simulink model "DDCU_wxt_v02_forA_LabviewV02"  (R2014a)
settings: Solver=FixedStepDiscrete  StartTime=0.0  StopTime=50  FixedStep=0.0005  RelTol=1e-3
InitFcn:
  | Veh_Par_wxt
values from neighbouring files (symbols this model uses):
  ag_thr = 0.4*g    (= 3.924)    [Veh_Par_wxt.m]
  B = 2.25    [Veh_Par_wxt.m]
  bra_pre_em = 12    [Veh_Par_wxt.m]
  bra_pre_gz2 = 12/3    (= 4)    [Veh_Par_wxt.m]
  bra_pre_gz34 = 12/3    (= 4)    [Veh_Par_wxt.m]
  bra_pre_yd = 12/2    (= 6)    [Veh_Par_wxt.m]
  brakepre_dem_data = [0 1 2 3 4 5 6 7 8 9 10 11 12]    [Veh_Par_wxt.m]
  brakeTrq_dem_data = [0 218.198 436.396 654.594 872.792 1090.99 1309.188 1527.386 1745.584 1963.782 2181.98 2400.178 2618.376]    [Veh_Par_wxt.m]
  bratrq_max = 4*2618.376    (= 10473.504)    [Veh_Par_wxt.m]
  eff_tran = 0.75    [Veh_Par_wxt.m]
  G = Mass*g    (= 36297)    [Veh_Par_wxt.m]
  kd1 = 1    [Veh_Par_wxt.m]
  kd2 = 1    [Veh_Par_wxt.m]
  kd3 = 1    [Veh_Par_wxt.m]
  ki1 = 1    [Veh_Par_wxt.m]
  ki2 = 1    [Veh_Par_wxt.m]
  ki3 = 1    [Veh_Par_wxt.m]
  kp1 = 1    [Veh_Par_wxt.m]
  kp2 = 1    [Veh_Par_wxt.m]
  kp3 = 1    [Veh_Par_wxt.m]
  L = 3.12    [Veh_Par_wxt.m]
  premax = 12    [Veh_Par_wxt.m]
  Radius = 0.20    (= 0.2)    [Veh_Par_wxt.m]
  s_opt_yi_add = 0.05    [Veh_Par_wxt.m]
  s_opt_zhuan_add = 0.05    [Veh_Par_wxt.m]
  spd_map_mot = [0 100 200 300 360 400 500 600 700 800 900]*tras_ratio    [Veh_Par_wxt.m]
  spdmax = 900*tras_ratio    (= 5580)    [Veh_Par_wxt.m]
  speed_thr_park = 5/3.6/Radius*30/pi    (= 66.3145596216)    [Veh_Par_wxt.m]
  tras_ratio = 6.2    [Veh_Par_wxt.m]
  trq_map_mot = [1200 1200 1200 1200 1200 1080 864 720 617 540 480]/tras_ratio    [Veh_Par_wxt.m]
  trqmax = 80    [Veh_Par_wxt.m]
  v_thr1_b = 5    [Veh_Par_wxt.m]
  v_thr2_b = 20    [Veh_Par_wxt.m]
  v_thr_park = 5    [Veh_Par_wxt.m]
undefined symbols (not defined in the file or in its folder): DiscIntNeverNeededParam
libraries: simulink x231, ec5744lib x19
(part 5 of 16)

== system DDCU_wxt_v02_forA_LabviewV02/Data_Input/MCU2_VCU3/MCU2_VCU3 ==
  input : Inport
  Enable : EnablePort
  Demux : Demux  Outputs=8
  M4Current_Ad : Sum
  M4Current_Convert : DataTypeConversion  OutDataTypeStr=uint32
  M4Current_F : Gain  Gain=0.5
  M4Current_L : simulink/Logic and Bit Operations/Bitwise Operator  logicop=AND  UseBitMask=on  BitMask=65520  BitMaskRealWorld=Stored Integer
  M4Current_O : Constant  Value=-600  OutDataTypeStr=single
  M4Current_S : ArithShift  BitShiftNumber=4
  M4Current_Sub : Subsystem
  M4Current_sat : Saturate  UpperLimit=1447.5  LowerLimit=-600
  M4Currentcv : DataTypeConversion
  M4Currentinput3_Ad : Sum
  M4Currentinput3_C : Constant  Value=256
  M4Currentinput3_P : Product
  M4Direction_Ad : Sum
  M4Direction_Convert : DataTypeConversion  OutDataTypeStr=uint32
  M4Direction_F : Gain
  M4Direction_L : simulink/Logic and Bit Operations/Bitwise Operator  logicop=AND  UseBitMask=on  BitMask=128  BitMaskRealWorld=Stored Integer
  M4Direction_O : Constant  Value=0  OutDataTypeStr=single
  M4Direction_S : ArithShift  BitShiftNumber=7
  M4Direction_Sub : Subsystem
  M4Direction_sat : Saturate  UpperLimit=1  LowerLimit=0
  M4Directioncv : DataTypeConversion
  M4HeartBeat_Ad : Sum
  M4HeartBeat_Convert : DataTypeConversion  OutDataTypeStr=uint32
  M4HeartBeat_F : Gain
  M4HeartBeat_L : simulink/Logic and Bit Operations/Bitwise Operator  logicop=AND  UseBitMask=on  BitMask=15  BitMaskRealWorld=Stored Integer
  M4HeartBeat_O : Constant  Value=0  OutDataTypeStr=single
  M4HeartBeat_S : ArithShift
  M4HeartBeat_Sub : Subsystem
  M4HeartBeat_sat : Saturate  UpperLimit=15  LowerLimit=0
  M4HeartBeatcv : DataTypeConversion
  M4InputVolt_Ad : Sum
  M4InputVolt_Convert : DataTypeConversion  OutDataTypeStr=uint32
  M4InputVolt_F : Gain  Gain=0.25
  M4InputVolt_L : simulink/Logic and Bit Operations/Bitwise Operator  logicop=AND  UseBitMask=on  BitMask=4095  BitMaskRealWorld=Stored Integer
  M4InputVolt_O : Constant  Value=0  OutDataTypeStr=single
  M4InputVolt_S : ArithShift
  M4InputVolt_Sub : Subsystem
  M4InputVolt_sat : Saturate  UpperLimit=1023.75  LowerLimit=0
  M4InputVoltcv : DataTypeConversion
  M4InputVoltinput8_Ad : Sum
  M4InputVoltinput8_C : Constant  Value=256
  M4InputVoltinput8_P : Product
  M4Speed_Ad : Sum
  M4Speed_Convert : DataTypeConversion  OutDataTypeStr=uint32
  M4Speed_F : Gain  Gain=5
  M4Speed_L : simulink/Logic and Bit Operations/Bitwise Operator  logicop=AND  UseBitMask=on  BitMask=65535  BitMaskRealWorld=Stored Integer
  M4Speed_O : Constant  Value=-5000  OutDataTypeStr=single
  M4Speed_S : ArithShift
  M4Speed_Sub : Subsystem
  M4Speed_sat : Saturate  UpperLimit=322675  LowerLimit=-5000
  M4Speedcv : DataTypeConversion
  M4Speedinput6_Ad : Sum
  M4Speedinput6_C : Constant  Value=256
  M4Speedinput6_P : Product
  M4State_Ad : Sum
  M4State_Convert : DataTypeConversion  OutDataTypeStr=uint32
  M4State_F : Gain
  M4State_L : simulink/Logic and Bit Operations/Bitwise Operator  logicop=AND  UseBitMask=on  BitMask=112  BitMaskRealWorld=Stored Integer
  M4State_O : Constant  Value=0  OutDataTypeStr=single
  M4State_S : ArithShift  BitShiftNumber=4
  M4State_Sub : Subsystem
  M4State_sat : Saturate  UpperLimit=7  LowerLimit=0
  M4Statecv : DataTypeConversion
  M4Torque_Ad : Sum
  M4Torque_Convert : DataTypeConversion  OutDataTypeStr=uint32
  M4Torque_F : Gain  Gain=0.25
  M4Torque_L : simulink/Logic and Bit Operations/Bitwise Operator  logicop=AND  UseBitMask=on  BitMask=4095  BitMaskRealWorld=Stored Integer
  M4Torque_O : Constant  Value=-300  OutDataTypeStr=single
  M4Torque_S : ArithShift
  M4Torque_Sub : Subsystem
  M4Torque_sat : Saturate  UpperLimit=723.75  LowerLimit=-300
  M4Torquecv : DataTypeConversion
  M4Torqueinput2_Ad : Sum
  M4Torqueinput2_C : Constant  Value=256
  M4Torqueinput2_P : Product
  M4InputVolt_Out : Outport
  M4Speed_Out : Outport  Port=2
  M4Direction_Out : Outport  Port=3
  M4State_Out : Outport  Port=4
  M4HeartBeat_Out : Outport  Port=5
  M4Current_Out : Outport  Port=6
  M4Torque_Out : Outport  Port=7
  wires:
  M4InputVolt_F/1 -> M4InputVolt_Ad/1
  M4InputVolt_O/1 -> M4InputVolt_Ad/2
  M4InputVolt_Ad/1 -> M4InputVolt_sat/1
  M4InputVolt_sat/1 -> M4InputVolt_Out/1
  Demux/8 -> M4InputVoltinput8_P/1
  M4InputVoltinput8_C/1 -> M4InputVoltinput8_P/2
  M4InputVoltinput8_P/1 -> M4InputVoltinput8_Ad/1
  Demux/7 -> M4InputVoltinput8_Ad/2
  M4InputVoltinput8_Ad/1 -> M4InputVolt_Sub/1(In1)
  M4InputVolt_Sub/1(Out1) -> M4InputVolt_Convert/1
  M4InputVolt_Convert/1 -> M4InputVolt_L/1
  M4InputVolt_L/1 -> M4InputVolt_S/1
  M4InputVolt_S/1 -> M4InputVoltcv/1
  M4InputVoltcv/1 -> M4InputVolt_F/1
  M4Speed_F/1 -> M4Speed_Ad/1
  M4Speed_O/1 -> M4Speed_Ad/2
  M4Speed_Ad/1 -> M4Speed_sat/1
  M4Speed_sat/1 -> M4Speed_Out/1
  Demux/6 -> M4Speedinput6_P/1
  M4Speedinput6_C/1 -> M4Speedinput6_P/2
  M4Speedinput6_P/1 -> M4Speedinput6_Ad/1
  Demux/5 -> M4Speedinput6_Ad/2
  M4Speedinput6_Ad/1 -> M4Speed_Sub/1(In1)
  M4Speed_Sub/1(Out1) -> M4Speed_Convert/1
  M4Speed_Convert/1 -> M4Speed_L/1
  M4Speed_L/1 -> M4Speed_S/1
  M4Speed_S/1 -> M4Speedcv/1
  M4Speedcv/1 -> M4Speed_F/1
  M4Direction_F/1 -> M4Direction_Ad/1
  M4Direction_O/1 -> M4Direction_Ad/2
  M4Direction_Ad/1 -> M4Direction_sat/1
  M4Direction_sat/1 -> M4Direction_Out/1
  Demux/4 -> M4State_Sub/1(In1), M4HeartBeat_Sub/1(In1), M4Direction_Sub/1(In1)
  M4Direction_Sub/1(Out1) -> M4Direction_Convert/1
  M4Direction_Convert/1 -> M4Direction_L/1
  M4Direction_L/1 -> M4Direction_S/1
  M4Direction_S/1 -> M4Directioncv/1
  M4Directioncv/1 -> M4Direction_F/1
  M4State_F/1 -> M4State_Ad/1
  M4State_O/1 -> M4State_Ad/2
  M4State_Ad/1 -> M4State_sat/1
  M4State_sat/1 -> M4State_Out/1
  M4State_Sub/1(Out1) -> M4State_Convert/1
  M4State_Convert/1 -> M4State_L/1
  M4State_L/1 -> M4State_S/1
  M4State_S/1 -> M4Statecv/1
  M4Statecv/1 -> M4State_F/1
  M4HeartBeat_F/1 -> M4HeartBeat_Ad/1
  M4HeartBeat_O/1 -> M4HeartBeat_Ad/2
  M4HeartBeat_Ad/1 -> M4HeartBeat_sat/1
  M4HeartBeat_sat/1 -> M4HeartBeat_Out/1
  M4HeartBeat_Sub/1(Out1) -> M4HeartBeat_Convert/1
  M4HeartBeat_Convert/1 -> M4HeartBeat_L/1
  M4HeartBeat_L/1 -> M4HeartBeat_S/1
  M4HeartBeat_S/1 -> M4HeartBeatcv/1
  M4HeartBeatcv/1 -> M4HeartBeat_F/1
  M4Current_F/1 -> M4Current_Ad/1
  M4Current_O/1 -> M4Current_Ad/2
  M4Current_Ad/1 -> M4Current_sat/1
  M4Current_sat/1 -> M4Current_Out/1
  Demux/3 -> M4Currentinput3_P/1
  M4Currentinput3_C/1 -> M4Currentinput3_P/2
  M4Currentinput3_P/1 -> M4Currentinput3_Ad/1
  Demux/2 -> M4Currentinput3_Ad/2, M4Torqueinput2_P/1
  M4Currentinput3_Ad/1 -> M4Current_Sub/1(In1)
  M4Current_Sub/1(Out1) -> M4Current_Convert/1
  M4Current_Convert/1 -> M4Current_L/1
  M4Current_L/1 -> M4Current_S/1
  M4Current_S/1 -> M4Currentcv/1
  M4Currentcv/1 -> M4Current_F/1
  M4Torque_F/1 -> M4Torque_Ad/1
  M4Torque_O/1 -> M4Torque_Ad/2
  M4Torque_Ad/1 -> M4Torque_sat/1
  M4Torque_sat/1 -> M4Torque_Out/1
  M4Torqueinput2_C/1 -> M4Torqueinput2_P/2
  M4Torqueinput2_P/1 -> M4Torqueinput2_Ad/1
  Demux/1 -> M4Torqueinput2_Ad/2
  M4Torqueinput2_Ad/1 -> M4Torque_Sub/1(In1)
  M4Torque_Sub/1(Out1) -> M4Torque_Convert/1
  M4Torque_Convert/1 -> M4Torque_L/1
  M4Torque_L/1 -> M4Torque_S/1
  M4Torque_S/1 -> M4Torquecv/1
  M4Torquecv/1 -> M4Torque_F/1
  input/1 -> Demux/1

== system DDCU_wxt_v02_forA_LabviewV02/Data_Input/MCU2_VCU4/MCU2_VCU4 ==
  input : Inport
  Enable : EnablePort
  Demux : Demux  Outputs=8
  M4FaultCode_Ad : Sum
  M4FaultCode_Convert : DataTypeConversion  OutDataTypeStr=uint32
  M4FaultCode_F : Gain
  M4FaultCode_L : simulink/Logic and Bit Operations/Bitwise Operator  logicop=AND  UseBitMask=on  BitMask=65520  BitMaskRealWorld=Stored Integer
  M4FaultCode_O : Constant  Value=0  OutDataTypeStr=single
  M4FaultCode_S : ArithShift  BitShiftNumber=4
  M4FaultCode_Sub : Subsystem
  M4FaultCode_sat : Saturate  UpperLimit=4095  LowerLimit=0
  M4FaultCodecv : DataTypeConversion
  M4FaultCodeinput8_Ad : Sum
  M4FaultCodeinput8_C : Constant  Value=256
  M4FaultCodeinput8_P : Product
  M4FaultGrade_Ad : Sum
  M4FaultGrade_Convert : DataTypeConversion  OutDataTypeStr=uint32
  M4FaultGrade_F : Gain
  M4FaultGrade_L : simulink/Logic and Bit Operations/Bitwise Operator  logicop=AND  UseBitMask=on  BitMask=15  BitMaskRealWorld=Stored Integer
  M4FaultGrade_O : Constant  Value=0  OutDataTypeStr=single
  M4FaultGrade_S : ArithShift
  M4FaultGrade_Sub : Subsystem
  M4FaultGrade_sat : Saturate  UpperLimit=15  LowerLimit=0
  M4FaultGradecv : DataTypeConversion
  M4IGBTTemp_Ad : Sum
  M4IGBTTemp_Convert : DataTypeConversion  OutDataTypeStr=uint32
  M4IGBTTemp_F : Gain
  M4IGBTTemp_L : simulink/Logic and Bit Operations/Bitwise Operator  logicop=AND  UseBitMask=on  BitMask=255  BitMaskRealWorld=Stored Integer
  M4IGBTTemp_O : Constant  Value=-50  OutDataTypeStr=single
  M4IGBTTemp_S : ArithShift
  M4IGBTTemp_Sub : Subsystem
  M4IGBTTemp_sat : Saturate  UpperLimit=205  LowerLimit=-50
  M4IGBTTempcv : DataTypeConversion
  M4Temp_Ad : Sum
  M4Temp_Convert : DataTypeConversion  OutDataTypeStr=uint32
  M4Temp_F : Gain
  M4Temp_L : simulink/Logic and Bit Operations/Bitwise Operator  logicop=AND  UseBitMask=on  BitMask=255  BitMaskRealWorld=Stored Integer
  M4Temp_O : Constant  Value=-50  OutDataTypeStr=single
  M4Temp_S : ArithShift
  M4Temp_Sub : Subsystem
  M4Temp_sat : Saturate  UpperLimit=205  LowerLimit=-50
  M4Tempcv : DataTypeConversion
  M4TqLimit_Ad : Sum
  M4TqLimit_Convert : DataTypeConversion  OutDataTypeStr=uint32
  M4TqLimit_F : Gain  Gain=0.125
  M4TqLimit_L : simulink/Logic and Bit Operations/Bitwise Operator  logicop=AND  UseBitMask=on  BitMask=65535  BitMaskRealWorld=Stored Integer
  M4TqLimit_O : Constant  Value=0  OutDataTypeStr=single
  M4TqLimit_S : ArithShift
  M4TqLimit_Sub : Subsystem
  M4TqLimit_sat : Saturate  UpperLimit=8191.875  LowerLimit=0
  M4TqLimitcv : DataTypeConversion
  M4TqLimitinput6_Ad : Sum
  M4TqLimitinput6_C : Constant  Value=256
  M4TqLimitinput6_P : Product
  M4FaultGrade_Out : Outport
  M4FaultCode_Out : Outport  Port=2
  M4TqLimit_Out : Outport  Port=3
  M4IGBTTemp_Out : Outport  Port=4
  M4Temp_Out : Outport  Port=5
  wires:
  M4FaultCode_F/1 -> M4FaultCode_Ad/1
  M4FaultCode_O/1 -> M4FaultCode_Ad/2
  M4FaultCode_Ad/1 -> M4FaultCode_sat/1
  M4FaultCode_sat/1 -> M4FaultCode_Out/1
  Demux/8 -> M4FaultCodeinput8_P/1
  M4FaultCodeinput8_C/1 -> M4FaultCodeinput8_P/2
  M4FaultCodeinput8_P/1 -> M4FaultCodeinput8_Ad/1
  Demux/7 -> M4FaultCodeinput8_Ad/2, M4FaultGrade_Sub/1(In1)
  M4FaultCodeinput8_Ad/1 -> M4FaultCode_Sub/1(In1)
  M4FaultCode_Sub/1(Out1) -> M4FaultCode_Convert/1
  M4FaultCode_Convert/1 -> M4FaultCode_L/1
  M4FaultCode_L/1 -> M4FaultCode_S/1
  M4FaultCode_S/1 -> M4FaultCodecv/1
  M4FaultCodecv/1 -> M4FaultCode_F/1
  M4FaultGrade_F/1 -> M4FaultGrade_Ad/1
  M4FaultGrade_O/1 -> M4FaultGrade_Ad/2
  M4FaultGrade_Ad/1 -> M4FaultGrade_sat/1
  M4FaultGrade_sat/1 -> M4FaultGrade_Out/1
  M4FaultGrade_Sub/1(Out1) -> M4FaultGrade_Convert/1
  M4FaultGrade_Convert/1 -> M4FaultGrade_L/1
  M4FaultGrade_L/1 -> M4FaultGrade_S/1
  M4FaultGrade_S/1 -> M4FaultGradecv/1
  M4FaultGradecv/1 -> M4FaultGrade_F/1
  M4TqLimit_F/1 -> M4TqLimit_Ad/1
  M4TqLimit_O/1 -> M4TqLimit_Ad/2
  M4TqLimit_Ad/1 -> M4TqLimit_sat/1
  M4TqLimit_sat/1 -> M4TqLimit_Out/1
  Demux/6 -> M4TqLimitinput6_P/1
  M4TqLimitinput6_C/1 -> M4TqLimitinput6_P/2
  M4TqLimitinput6_P/1 -> M4TqLimitinput6_Ad/1
  Demux/5 -> M4TqLimitinput6_Ad/2
  M4TqLimitinput6_Ad/1 -> M4TqLimit_Sub/1(In1)
  M4TqLimit_Sub/1(Out1) -> M4TqLimit_Convert/1
  M4TqLimit_Convert/1 -> M4TqLimit_L/1
  M4TqLimit_L/1 -> M4TqLimit_S/1
  M4TqLimit_S/1 -> M4TqLimitcv/1
  M4TqLimitcv/1 -> M4TqLimit_F/1
  M4IGBTTemp_F/1 -> M4IGBTTemp_Ad/1
  M4IGBTTemp_O/1 -> M4IGBTTemp_Ad/2
  M4IGBTTemp_Ad/1 -> M4IGBTTemp_sat/1
  M4IGBTTemp_sat/1 -> M4IGBTTemp_Out/1
  Demux/2 -> M4IGBTTemp_Sub/1(In1)
  M4IGBTTemp_Sub/1(Out1) -> M4IGBTTemp_Convert/1
  M4IGBTTemp_Convert/1 -> M4IGBTTemp_L/1
  M4IGBTTemp_L/1 -> M4IGBTTemp_S/1
  M4IGBTTemp_S/1 -> M4IGBTTempcv/1
  M4IGBTTempcv/1 -> M4IGBTTemp_F/1
  M4Temp_F/1 -> M4Temp_Ad/1
  M4Temp_O/1 -> M4Temp_Ad/2
  M4Temp_Ad/1 -> M4Temp_sat/1
  M4Temp_sat/1 -> M4Temp_Out/1
  Demux/1 -> M4Temp_Sub/1(In1)
  M4Temp_Sub/1(Out1) -> M4Temp_Convert/1
  M4Temp_Convert/1 -> M4Temp_L/1
  M4Temp_L/1 -> M4Temp_S/1
  M4Temp_S/1 -> M4Tempcv/1
  M4Tempcv/1 -> M4Temp_F/1
  input/1 -> Demux/1

== system DDCU_wxt_v02_forA_LabviewV02/MainControl/mode_control/Park ==
  Signals : Inport
  Action Port : ActionPort  ActionType=case
  Mux : Mux  Inputs=6
  park : Subsystem
  park_dem : Outport
  wires:
  Signals/1 -> park/1(Signals)
  park/4(mot_rr) -> Mux/4
  park/3(mot_rf) -> Mux/3
  park/5(bra_pre_l) -> Mux/5
  park/2(mot_lr) -> Mux/2
  park/6(bra_pre_r) -> Mux/6
  park/1(mot_lf) -> Mux/1
  Mux/1 -> park_dem/1

== system DDCU_wxt_v02_forA_LabviewV02/MainControl/mode_control/backward ==
  Signals : Inport
  Action Port : ActionPort  ActionType=case
  backward : Subsystem
  backward_dem : Outport
  wires:
  Signals/1 -> backward/1(Signals)
  backward/1(backward_dem) -> backward_dem/1

== system DDCU_wxt_v02_forA_LabviewV02/MainControl/mode_control/center_steer ==
  Signals : Inport
  Action Port : ActionPort  ActionType=case
  Mux : Mux  Inputs=6
  center_steer : Subsystem
  center_steer_dem : Outport
  wires:
  Mux/1 -> center_steer_dem/1
  center_steer/6(bra_pre_r) -> Mux/6
  center_steer/5(bra_pre_l) -> Mux/5
  Signals/1 -> center_steer/1(Signals)
  center_steer/1(mot_lf) -> Mux/1
  center_steer/2(mot_lr) -> Mux/2
  center_steer/4(mot_rr) -> Mux/4
  center_steer/3(mot_rf) -> Mux/3

== system DDCU_wxt_v02_forA_LabviewV02/MainControl/mode_control/emergency_stop ==
  Signals : Inport
  Action Port : ActionPort  ActionType=case
  Mux : Mux  Inputs=6
  emergency_stop : Subsystem
  emergency_stop_dem : Outport
  wires:
  Mux/1 -> emergency_stop_dem/1
  emergency_stop/1(mot_lf) -> Mux/1
  emergency_stop/6(bra_pre_r) -> Mux/6
  emergency_stop/4(mot_rr) -> Mux/4
  emergency_stop/5(bra_pre_l) -> Mux/5
  emergency_stop/3(mot_rf) -> Mux/3
  emergency_stop/2(mot_lr) -> Mux/2
  Signals/1 -> emergency_stop/1(Signals)

== system DDCU_wxt_v02_forA_LabviewV02/MainControl/mode_control/forward ==
  Signals : Inport
  Action Port : ActionPort  ActionType=case
  forward : Subsystem
  forward_dem : Outport
  wires:
  forward/1(forward_dem) -> forward_dem/1
  Signals/1 -> forward/1(Signals)

== system DDCU_wxt_v02_forA_LabviewV02/MainControl/mode_control/neutral ==
  Signals : Inport
  Action Port : ActionPort  ActionType=case
  Mux : Mux  Inputs=6
  neutral : Subsystem
  neutral_dem : Outport
  wires:
  Mux/1 -> neutral_dem/1
  Signals/1 -> neutral/1(Signals)
  neutral/2(mot_lr) -> Mux/2
  neutral/3(mot_rf) -> Mux/3
  neutral/1(mot_lf) -> Mux/1
  neutral/6(bra_pre_r) -> Mux/6
  neutral/5(bra_pre_l) -> Mux/5
  neutral/4(mot_rr) -> Mux/4

== system DDCU_wxt_v02_forA_LabviewV02/OutputSignalProcess/VCU_ESC/VVMS_BrkPSetLe_MPa ==
  VVMS_BrkPSetLe_MPa : Inport
  Constant{2..8} (7 alike) : Constant  Value=0  OutDataTypeStr=uint8
  VVMS_BrkPSetLe_MPaRon : Rounding  Operator=round
  VVMS_BrkPSetLe_MPa_1sat : Saturate  UpperLimit=255  LowerLimit=0
  VVMS_BrkPSetLe_MPa_Convert : DataTypeConversion  OutDataTypeStr=uint8
  VVMS_BrkPSetLe_MPa_Convert1 : DataTypeConversion  OutDataTypeStr=uint32
  VVMS_BrkPSetLe_MPa_D : Product  Inputs=*/
  VVMS_BrkPSetLe_MPa_F : Constant  Value=0.1  OutDataTypeStr=single
  VVMS_BrkPSetLe_MPa_L : simulink/Logic and Bit Operations/Bitwise Operator  logicop=AND  UseBitMask=on  BitMask=255  BitMaskRealWorld=Stored Integer
  VVMS_BrkPSetLe_MPa_O : Constant  Value=0  OutDataTypeStr=single
  VVMS_BrkPSetLe_MPa_S : ArithShift
  VVMS_BrkPSetLe_MPa_sat : Saturate  UpperLimit=25.5  LowerLimit=0
  VVMS_BrkPSetLe_MPa_st : Sum  Inputs=+-
  output1 : Outport
  output2 : Outport  Port=2
  output3 : Outport  Port=3
  output4 : Outport  Port=4
  output5 : Outport  Port=5
  output6 : Outport  Port=6
  output7 : Outport  Port=7
  output8 : Outport  Port=8
  wires:
  VVMS_BrkPSetLe_MPa/1 -> VVMS_BrkPSetLe_MPa_sat/1
  VVMS_BrkPSetLe_MPa_sat/1 -> VVMS_BrkPSetLe_MPa_st/1
  VVMS_BrkPSetLe_MPa_O/1 -> VVMS_BrkPSetLe_MPa_st/2
  VVMS_BrkPSetLe_MPa_st/1 -> VVMS_BrkPSetLe_MPa_D/1
  VVMS_BrkPSetLe_MPa_F/1 -> VVMS_BrkPSetLe_MPa_D/2
  VVMS_BrkPSetLe_MPa_D/1 -> VVMS_BrkPSetLe_MPaRon/1
  VVMS_BrkPSetLe_MPaRon/1 -> VVMS_BrkPSetLe_MPa_S/1
  VVMS_BrkPSetLe_MPa_S/1 -> VVMS_BrkPSetLe_MPa_1sat/1
  VVMS_BrkPSetLe_MPa_1sat/1 -> VVMS_BrkPSetLe_MPa_Convert1/1
  VVMS_BrkPSetLe_MPa_Convert1/1 -> VVMS_BrkPSetLe_MPa_L/1
  VVMS_BrkPSetLe_MPa_L/1 -> VVMS_BrkPSetLe_MPa_Convert/1
  VVMS_BrkPSetLe_MPa_Convert/1 -> output1/1
  Constant2/1 -> output2/1
  Constant3/1 -> output3/1
  Constant4/1 -> output4/1
  Constant5/1 -> output5/1
  Constant6/1 -> output6/1
  Constant7/1 -> output7/1
  Constant8/1 -> output8/1

== system DDCU_wxt_v02_forA_LabviewV02/OutputSignalProcess/VCU_ESC/VVMS_BrkPSetRi_MPa ==
  VVMS_BrkPSetRi_MPa : Inport
  Constant{1,3..8} (7 alike) : Constant  Value=0  OutDataTypeStr=uint8
  VVMS_BrkPSetRi_MPaRon : Rounding  Operator=round
  VVMS_BrkPSetRi_MPa_1sat : Saturate  UpperLimit=255  LowerLimit=0
  VVMS_BrkPSetRi_MPa_Convert : DataTypeConversion  OutDataTypeStr=uint8
  VVMS_BrkPSetRi_MPa_Convert1 : DataTypeConversion  OutDataTypeStr=uint32
  VVMS_BrkPSetRi_MPa_D : Product  Inputs=*/
  VVMS_BrkPSetRi_MPa_F : Constant  Value=0.1  OutDataTypeStr=single
  VVMS_BrkPSetRi_MPa_L : simulink/Logic and Bit Operations/Bitwise Operator  logicop=AND  UseBitMask=on  BitMask=255  BitMaskRealWorld=Stored Integer
  VVMS_BrkPSetRi_MPa_O : Constant  Value=0  OutDataTypeStr=single
  VVMS_BrkPSetRi_MPa_S : ArithShift
  VVMS_BrkPSetRi_MPa_sat : Saturate  UpperLimit=25.5  LowerLimit=0
  VVMS_BrkPSetRi_MPa_st : Sum  Inputs=+-
  output1 : Outport
  output2 : Outport  Port=2
  output3 : Outport  Port=3
  output4 : Outport  Port=4
  output5 : Outport  Port=5
  output6 : Outport  Port=6
  output7 : Outport  Port=7
  output8 : Outport  Port=8
  wires:
  VVMS_BrkPSetRi_MPa/1 -> VVMS_BrkPSetRi_MPa_sat/1
  VVMS_BrkPSetRi_MPa_sat/1 -> VVMS_BrkPSetRi_MPa_st/1
  VVMS_BrkPSetRi_MPa_O/1 -> VVMS_BrkPSetRi_MPa_st/2
  VVMS_BrkPSetRi_MPa_st/1 -> VVMS_BrkPSetRi_MPa_D/1
  VVMS_BrkPSetRi_MPa_F/1 -> VVMS_BrkPSetRi_MPa_D/2
  VVMS_BrkPSetRi_MPa_D/1 -> VVMS_BrkPSetRi_MPaRon/1
  VVMS_BrkPSetRi_MPaRon/1 -> VVMS_BrkPSetRi_MPa_S/1
  VVMS_BrkPSetRi_MPa_S/1 -> VVMS_BrkPSetRi_MPa_1sat/1
  VVMS_BrkPSetRi_MPa_1sat/1 -> VVMS_BrkPSetRi_MPa_Convert1/1
  VVMS_BrkPSetRi_MPa_Convert1/1 -> VVMS_BrkPSetRi_MPa_L/1
  VVMS_BrkPSetRi_MPa_L/1 -> VVMS_BrkPSetRi_MPa_Convert/1
  VVMS_BrkPSetRi_MPa_Convert/1 -> output2/1
  Constant1/1 -> output1/1
  Constant3/1 -> output3/1
  Constant4/1 -> output4/1
  Constant5/1 -> output5/1
  Constant6/1 -> output6/1
  Constant7/1 -> output7/1
  Constant8/1 -> output8/1

== system DDCU_wxt_v02_forA_LabviewV02/OutputSignalProcess/VCU_ESC/VVMS_BrkSts_flg ==
  VVMS_BrkSts_flg : Inport
  Constant{1..2,4..8} (7 alike) : Constant  Value=0  OutDataTypeStr=uint8
  VVMS_BrkSts_flgRon : Rounding  Operator=round
  VVMS_BrkSts_flg_1sat : Saturate  UpperLimit=64  LowerLimit=0
  VVMS_BrkSts_flg_Convert : DataTypeConversion  OutDataTypeStr=uint8
  VVMS_BrkSts_flg_Convert1 : DataTypeConversion  OutDataTypeStr=uint32
  VVMS_BrkSts_flg_D : Product  Inputs=*/
  VVMS_BrkSts_flg_F : Constant  OutDataTypeStr=single
  VVMS_BrkSts_flg_L : simulink/Logic and Bit Operations/Bitwise Operator  logicop=AND  UseBitMask=on  BitMask=64  BitMaskRealWorld=Stored Integer
  VVMS_BrkSts_flg_O : Constant  Value=0  OutDataTypeStr=single
  VVMS_BrkSts_flg_S : ArithShift  BitShiftNumber=-6
  VVMS_BrkSts_flg_sat : Saturate  UpperLimit=1  LowerLimit=0
  VVMS_BrkSts_flg_st : Sum  Inputs=+-
  output1 : Outport
  output2 : Outport  Port=2
  output3 : Outport  Port=3
  output4 : Outport  Port=4
  output5 : Outport  Port=5
  output6 : Outport  Port=6
  output7 : Outport  Port=7
  output8 : Outport  Port=8
  wires:
  VVMS_BrkSts_flg/1 -> VVMS_BrkSts_flg_sat/1
  VVMS_BrkSts_flg_sat/1 -> VVMS_BrkSts_flg_st/1
  VVMS_BrkSts_flg_O/1 -> VVMS_BrkSts_flg_st/2
  VVMS_BrkSts_flg_st/1 -> VVMS_BrkSts_flg_D/1
  VVMS_BrkSts_flg_F/1 -> VVMS_BrkSts_flg_D/2
  VVMS_BrkSts_flg_D/1 -> VVMS_BrkSts_flgRon/1
  VVMS_BrkSts_flgRon/1 -> VVMS_BrkSts_flg_S/1
  VVMS_BrkSts_flg_S/1 -> VVMS_BrkSts_flg_1sat/1
  VVMS_BrkSts_flg_1sat/1 -> VVMS_BrkSts_flg_Convert1/1
  VVMS_BrkSts_flg_Convert1/1 -> VVMS_BrkSts_flg_L/1
  VVMS_BrkSts_flg_L/1 -> VVMS_BrkSts_flg_Convert/1
  VVMS_BrkSts_flg_Convert/1 -> output3/1
  Constant1/1 -> output1/1
  Constant2/1 -> output2/1
  Constant4/1 -> output4/1
  Constant5/1 -> output5/1
  Constant6/1 -> output6/1
  Constant7/1 -> output7/1
  Constant8/1 -> output8/1

== system DDCU_wxt_v02_forA_LabviewV02/OutputSignalProcess/VCU_ESC/VVMS_ParkSts_flg ==
  VVMS_ParkSts_flg : Inport
  Constant{1..2,4..8} (7 alike) : Constant  Value=0  OutDataTypeStr=uint8
  VVMS_ParkSts_flgRon : Rounding  Operator=round
  VVMS_ParkSts_flg_1sat : Saturate  UpperLimit=128  LowerLimit=0
  VVMS_ParkSts_flg_Convert : DataTypeConversion  OutDataTypeStr=uint8
  VVMS_ParkSts_flg_Convert1 : DataTypeConversion  OutDataTypeStr=uint32
  VVMS_ParkSts_flg_D : Product  Inputs=*/
  VVMS_ParkSts_flg_F : Constant  OutDataTypeStr=single
  VVMS_ParkSts_flg_L : simulink/Logic and Bit Operations/Bitwise Operator  logicop=AND  UseBitMask=on  BitMask=128  BitMaskRealWorld=Stored Integer
  VVMS_ParkSts_flg_O : Constant  Value=0  OutDataTypeStr=single
  VVMS_ParkSts_flg_S : ArithShift  BitShiftNumber=-7
  VVMS_ParkSts_flg_sat : Saturate  UpperLimit=1  LowerLimit=0
  VVMS_ParkSts_flg_st : Sum  Inputs=+-
  output1 : Outport
  output2 : Outport  Port=2
  output3 : Outport  Port=3
  output4 : Outport  Port=4
  output5 : Outport  Port=5
  output6 : Outport  Port=6
  output7 : Outport  Port=7
  output8 : Outport  Port=8
  wires:
  VVMS_ParkSts_flg/1 -> VVMS_ParkSts_flg_sat/1
  VVMS_ParkSts_flg_sat/1 -> VVMS_ParkSts_flg_st/1
  VVMS_ParkSts_flg_O/1 -> VVMS_ParkSts_flg_st/2
  VVMS_ParkSts_flg_st/1 -> VVMS_ParkSts_flg_D/1
  VVMS_ParkSts_flg_F/1 -> VVMS_ParkSts_flg_D/2
  VVMS_ParkSts_flg_D/1 -> VVMS_ParkSts_flgRon/1
  VVMS_ParkSts_flgRon/1 -> VVMS_ParkSts_flg_S/1
  VVMS_ParkSts_flg_S/1 -> VVMS_ParkSts_flg_1sat/1
  VVMS_ParkSts_flg_1sat/1 -> VVMS_ParkSts_flg_Convert1/1
  VVMS_ParkSts_flg_Convert1/1 -> VVMS_ParkSts_flg_L/1
  VVMS_ParkSts_flg_L/1 -> VVMS_ParkSts_flg_Convert/1
  VVMS_ParkSts_flg_Convert/1 -> output3/1
  Constant1/1 -> output1/1
  Constant2/1 -> output2/1
  Constant4/1 -> output4/1
  Constant5/1 -> output5/1
  Constant6/1 -> output6/1
  Constant7/1 -> output7/1
  Constant8/1 -> output8/1

== matlab function DDCU_wxt_v02_forA_LabviewV02/MainControl/mode_control/backward/backward/Brake/MATLAB Function ==
  data: guzhang_lf input; gz_total output; guzhang_lr input; guzhang_rf input; guzhang_rr input
function gz_total = fcn(guzhang_lf,guzhang_lr,guzhang_rf,guzhang_rr)
%#codegen
if guzhang_lf==0 && guzhang_lr==0 && guzhang_rf==0 && guzhang_rr==0
    gz_total=0;
else
    gz_total=1;
end
end

== matlab function DDCU_wxt_v02_forA_LabviewV02/MainControl/mode_control/backward/backward/Brake/MATLAB Function2 ==
  data: syi_act_lr input; flagyi_lr output; s_opt_yi input; s_opt_yi_add input; flagyi_lr_pre input
function flagyi_lr = fcn(syi_act_lr,s_opt_yi,s_opt_yi_add,flagyi_lr_pre)
%#codegen
if syi_act_lr>s_opt_yi+s_opt_yi_add
    flagyi_lr=1;
elseif syi_act_lr<s_opt_yi
    flagyi_lr = 0;
else
    flagyi_lr=flagyi_lr_pre;
end
end

== matlab function DDCU_wxt_v02_forA_LabviewV02/MainControl/mode_control/backward/backward/Drive/MATLAB Function ==
  data: acc_y input; y output; steer_dem input; ag_thr input
function y = fcn(acc_y,steer_dem,ag_thr)
%#codegen
if abs(acc_y)>=ag_thr
    y=0;
elseif steer_dem~=0
    y=1;
else 
    y=2;
end
end

== matlab function DDCU_wxt_v02_forA_LabviewV02/MainControl/mode_control/backward/backward/Drive/驱动防滑控制TCS/MATLAB Function ==
  data: steer_dem input; y output
function y = fcn(steer_dem)
%#codegen 如果有转向，y=0,无转向，y=1
if steer_dem~=0
y = 0;
else y=1;
end
end

== matlab function DDCU_wxt_v02_forA_LabviewV02/MainControl/mode_control/backward/backward/Drive/驱动防滑控制TCS/直行TCS/直行/MATLAB Function1 ==
  data: s_act_lr input; flag_lr output; s_opt_zhuan input; s_opt_zhuan_add input; flag_lr_pre input
function flag_lr = fcn(s_act_lr,s_opt_zhuan,s_opt_zhuan_add,flag_lr_pre)
%#codegen
if s_act_lr>s_opt_zhuan+s_opt_zhuan_add
    flag_lr=1;
elseif s_act_lr<s_opt_zhuan
    flag_lr = 0;
else
    flag_lr=flag_lr_pre;
end
end

== matlab function DDCU_wxt_v02_forA_LabviewV02/MainControl/mode_control/backward/backward/Drive/驱动防滑控制TCS/转向TCS/右转/MATLAB Function2 ==
  data: s_act_rf input; flag_rf output; s_opt_zhuan input; s_opt_zhuan_add input; flag_rf_pre input
function flag_rf = fcn(s_act_rf,s_opt_zhuan,s_opt_zhuan_add,flag_rf_pre)
%#codegen
if s_act_rf>s_opt_zhuan+s_opt_zhuan_add
    flag_rf=1;
elseif s_act_rf<s_opt_zhuan
    flag_rf = 0;
else
    flag_rf=flag_rf_pre;
end
end

== matlab function DDCU_wxt_v02_forA_LabviewV02/MainControl/mode_control/backward/backward/Drive/驱动防滑控制TCS/转向TCS/右转/后轮滑转/HeartBeat ==
  data: life_pre input; life output
function life = fcn(life_pre)
%#codegen
life=life_pre+1;
if life>15
    life=0;
end
end

== matlab function DDCU_wxt_v02_forA_LabviewV02/MainControl/mode_control/backward/backward/Drive/驱动防滑控制TCS/转向TCS/左转/MATLAB Function2 ==
  data: s_act_rf input; flag_rf output; s_opt_zhuan input; s_opt_zhuan_add input; flag_rf_pre input
function flag_rf = fcn(s_act_rf,s_opt_zhuan,s_opt_zhuan_add,flag_rf_pre)
%#codegen
if s_act_rf>s_opt_zhuan+s_opt_zhuan_add
    flag_rf=1;
elseif s_act_rf<s_opt_zhuan
    flag_rf = 0;
else
    flag_rf=flag_rf_pre;
end
end

== matlab function DDCU_wxt_v02_forA_LabviewV02/MainControl/mode_control/backward/backward/Drive/驱动防滑控制TCS/转向TCS/左转/前轮滑转/HeartBeat1 ==
  data: life_pre input; life output
function life = fcn(life_pre)
%#codegen
life=life_pre+1;
if life>15
    life=0;
end
end

== matlab function DDCU_wxt_v02_forA_LabviewV02/MainControl/mode_control/backward/backward/MATLAB Function ==
  data: acc_dem input; y output; brake_dem input; HAC input
function y = fcn(acc_dem,brake_dem,HAC)
%#codegen
if HAC==1
    if acc_dem>0
        y=0;
    else
        y=1;
    end
else
    if brake_dem==0
        y=0;
    else
        y=1;
    end
end
end

== system DDCU_wxt_v02_forA_LabviewV02/OutputSignalProcess/VCU_MCU1/M1Drive ==
  M1Drive : Inport
  Constant{2..8} (7 alike) : Constant  Value=0  OutDataTypeStr=uint8
  M1DriveRon : Rounding  Operator=round
  M1Drive_1sat : Saturate  UpperLimit=48  LowerLimit=0
  M1Drive_Convert : DataTypeConversion  OutDataTypeStr=uint8
  M1Drive_Convert1 : DataTypeConversion  OutDataTypeStr=uint32
  M1Drive_D : Product  Inputs=*/
  M1Drive_F : Constant  OutDataTypeStr=single
  M1Drive_L : simulink/Logic and Bit Operations/Bitwise Operator  logicop=AND  UseBitMask=on  BitMask=48  BitMaskRealWorld=Stored Integer
  M1Drive_O : Constant  Value=0  OutDataTypeStr=single
  M1Drive_S : ArithShift  BitShiftNumber=-4
  M1Drive_sat : Saturate  UpperLimit=3  LowerLimit=0
  M1Drive_st : Sum  Inputs=+-
  output1 : Outport
  output2 : Outport  Port=2
  output3 : Outport  Port=3
  output4 : Outport  Port=4
  output5 : Outport  Port=5
  output6 : Outport  Port=6
  output7 : Outport  Port=7
  output8 : Outport  Port=8
  wires:
  M1Drive/1 -> M1Drive_sat/1
  M1Drive_sat/1 -> M1Drive_st/1
  M1Drive_O/1 -> M1Drive_st/2
  M1Drive_st/1 -> M1Drive_D/1
  M1Drive_F/1 -> M1Drive_D/2
  M1Drive_D/1 -> M1DriveRon/1
  M1DriveRon/1 -> M1Drive_S/1
  M1Drive_S/1 -> M1Drive_1sat/1
  M1Drive_1sat/1 -> M1Drive_Convert1/1
  M1Drive_Convert1/1 -> M1Drive_L/1
  M1Drive_L/1 -> M1Drive_Convert/1
  M1Drive_Convert/1 -> output1/1
  Constant2/1 -> output2/1
  Constant3/1 -> output3/1
  Constant4/1 -> output4/1
  Constant5/1 -> output5/1
  Constant6/1 -> output6/1
  Constant7/1 -> output7/1
  Constant8/1 -> output8/1

== system DDCU_wxt_v02_forA_LabviewV02/OutputSignalProcess/VCU_MCU1/M1Enable ==
  M1Enable : Inport
  Constant{2..8} (7 alike) : Constant  Value=0  OutDataTypeStr=uint8
  M1EnableRon : Rounding  Operator=round
  M1Enable_1sat : Saturate  UpperLimit=3  LowerLimit=0
  M1Enable_Convert : DataTypeConversion  OutDataTypeStr=uint8
  M1Enable_Convert1 : DataTypeConversion  OutDataTypeStr=uint32
  M1Enable_D : Product  Inputs=*/
  M1Enable_F : Constant  OutDataTypeStr=single
  M1Enable_L : simulink/Logic and Bit Operations/Bitwise Operator  logicop=AND  UseBitMask=on  BitMask=3  BitMaskRealWorld=Stored Integer
  M1Enable_O : Constant  Value=0  OutDataTypeStr=single
  M1Enable_S : ArithShift
  M1Enable_sat : Saturate  UpperLimit=3  LowerLimit=0
  M1Enable_st : Sum  Inputs=+-
  output1 : Outport
  output2 : Outport  Port=2
  output3 : Outport  Port=3
  output4 : Outport  Port=4
  output5 : Outport  Port=5
  output6 : Outport  Port=6
  output7 : Outport  Port=7
  output8 : Outport  Port=8
  wires:
  M1Enable/1 -> M1Enable_sat/1
  M1Enable_sat/1 -> M1Enable_st/1
  M1Enable_O/1 -> M1Enable_st/2
  M1Enable_st/1 -> M1Enable_D/1
  M1Enable_F/1 -> M1Enable_D/2
  M1Enable_D/1 -> M1EnableRon/1
  M1EnableRon/1 -> M1Enable_S/1
  M1Enable_S/1 -> M1Enable_1sat/1
  M1Enable_1sat/1 -> M1Enable_Convert1/1
  M1Enable_Convert1/1 -> M1Enable_L/1
  M1Enable_L/1 -> M1Enable_Convert/1
  M1Enable_Convert/1 -> output1/1
  Constant2/1 -> output2/1
  Constant3/1 -> output3/1
  Constant4/1 -> output4/1
  Constant5/1 -> output5/1
  Constant6/1 -> output6/1
  Constant7/1 -> output7/1
  Constant8/1 -> output8/1

== system DDCU_wxt_v02_forA_LabviewV02/OutputSignalProcess/VCU_MCU1/M1Mode ==
  M1Mode : Inport
  Constant{2..8} (7 alike) : Constant  Value=0  OutDataTypeStr=uint8
  M1ModeRon : Rounding  Operator=round
  M1Mode_1sat : Saturate  UpperLimit=12  LowerLimit=0
  M1Mode_Convert : DataTypeConversion  OutDataTypeStr=uint8
  M1Mode_Convert1 : DataTypeConversion  OutDataTypeStr=uint32
  M1Mode_D : Product  Inputs=*/
  M1Mode_F : Constant  OutDataTypeStr=single
  M1Mode_L : simulink/Logic and Bit Operations/Bitwise Operator  logicop=AND  UseBitMask=on  BitMask=12  BitMaskRealWorld=Stored Integer
  M1Mode_O : Constant  Value=0  OutDataTypeStr=single
  M1Mode_S : ArithShift  BitShiftNumber=-2
  M1Mode_sat : Saturate  UpperLimit=3  LowerLimit=0
  M1Mode_st : Sum  Inputs=+-
  output1 : Outport
  output2 : Outport  Port=2
  output3 : Outport  Port=3
  output4 : Outport  Port=4
  output5 : Outport  Port=5
  output6 : Outport  Port=6
  output7 : Outport  Port=7
  output8 : Outport  Port=8
  wires:
  M1Mode/1 -> M1Mode_sat/1
  M1Mode_sat/1 -> M1Mode_st/1
  M1Mode_O/1 -> M1Mode_st/2
  M1Mode_st/1 -> M1Mode_D/1
  M1Mode_F/1 -> M1Mode_D/2
  M1Mode_D/1 -> M1ModeRon/1
  M1ModeRon/1 -> M1Mode_S/1
  M1Mode_S/1 -> M1Mode_1sat/1
  M1Mode_1sat/1 -> M1Mode_Convert1/1
  M1Mode_Convert1/1 -> M1Mode_L/1
  M1Mode_L/1 -> M1Mode_Convert/1
  M1Mode_Convert/1 -> output1/1
  Constant2/1 -> output2/1
  Constant3/1 -> output3/1
  Constant4/1 -> output4/1
  Constant5/1 -> output5/1
  Constant6/1 -> output6/1
  Constant7/1 -> output7/1
  Constant8/1 -> output8/1

== system DDCU_wxt_v02_forA_LabviewV02/OutputSignalProcess/VCU_MCU1/M1SpeedLimit ==
  M1SpeedLimit : Inport
  BitCov : DataTypeConversion  OutDataTypeStr=uint8
  Constant{1..2,5..8} (6 alike) : Constant  Value=0  OutDataTypeStr=uint8
  M1SpeedLimitCOV : DataTypeConversion  OutDataTypeStr=uint8
  M1SpeedLimitRon : Rounding  Operator=round
  M1SpeedLimit_1sat : Saturate  UpperLimit=16380  LowerLimit=0
  M1SpeedLimit_And : simulink/Logic and Bit Operations/Bitwise Operator  logicop=AND  UseBitMask=off  NumInputPorts=2  BitMask=bin2dec('11011001')  BitMaskRealWorld=Stored Integer
  M1SpeedLimit_And_C : Constant  Value=255  OutDataTypeStr=uint32
  M1SpeedLimit_Convert : DataTypeConversion  OutDataTypeStr=uint32
  M1SpeedLimit_D : Product  Inputs=*/
  M1SpeedLimit_D1 : Product  Inputs=*/
  M1SpeedLimit_F : Constant  Value=5  OutDataTypeStr=single
  M1SpeedLimit_L : simulink/Logic and Bit Operations/Bitwise Operator  logicop=AND  UseBitMask=on  BitMask=16380  BitMaskRealWorld=Stored Integer
  M1SpeedLimit_O : Constant  Value=0  OutDataTypeStr=single
  M1SpeedLimit_S : ArithShift  BitShiftNumber=-2
  M1SpeedLimit_sat : Saturate  UpperLimit=20475  LowerLimit=0
  M1SpeedLimit_st : Sum  Inputs=+-
  M1SpeedLimitoutput4_C : Constant  Value=256
  output1 : Outport
  output2 : Outport  Port=2
  output3 : Outport  Port=3
  output4 : Outport  Port=4
  output5 : Outport  Port=5
  output6 : Outport  Port=6
  output7 : Outport  Port=7
  output8 : Outport  Port=8
  wires:
  M1SpeedLimit/1 -> M1SpeedLimit_sat/1
  M1SpeedLimit_sat/1 -> M1SpeedLimit_st/1
  M1SpeedLimit_O/1 -> M1SpeedLimit_st/2
  M1SpeedLimit_st/1 -> M1SpeedLimit_D/1
  M1SpeedLimit_F/1 -> M1SpeedLimit_D/2
  M1SpeedLimit_D/1 -> M1SpeedLimitRon/1
  M1SpeedLimitRon/1 -> M1SpeedLimit_S/1
  M1SpeedLimit_S/1 -> M1SpeedLimit_1sat/1
  M1SpeedLimit_1sat/1 -> M1SpeedLimit_Convert/1
  M1SpeedLimit_Convert/1 -> M1SpeedLimit_L/1
  M1SpeedLimit_L/1 -> M1SpeedLimit_D1/1, M1SpeedLimit_And/1
  M1SpeedLimitoutput4_C/1 -> M1SpeedLimit_D1/2
  M1SpeedLimit_D1/1 -> M1SpeedLimitCOV/1
  M1SpeedLimitCOV/1 -> output4/1
  M1SpeedLimit_And_C/1 -> M1SpeedLimit_And/2
  M1SpeedLimit_And/1 -> BitCov/1
  BitCov/1 -> output3/1
  Constant1/1 -> output1/1
  Constant2/1 -> output2/1
  Constant5/1 -> output5/1
  Constant6/1 -> output6/1
  Constant7/1 -> output7/1
  Constant8/1 -> output8/1

== system DDCU_wxt_v02_forA_LabviewV02/OutputSignalProcess/VCU_MCU1/M1TorqueSet ==
  M1TorqueSet : Inport
  Constant{4..8} (5 alike) : Constant  Value=0  OutDataTypeStr=uint8
  M1TorqueSetBitCov : DataTypeConversion  OutDataTypeStr=uint32
  M1TorqueSetBitCov1 : DataTypeConversion  OutDataTypeStr=uint8
  M1TorqueSetCOV : DataTypeConversion  OutDataTypeStr=uint8
  M1TorqueSetCOV1 : DataTypeConversion  OutDataTypeStr=uint8
  M1TorqueSetRon : Rounding  Operator=round
  M1TorqueSet_1sat : Saturate  UpperLimit=262080  LowerLimit=0
  M1TorqueSet_And : simulink/Logic and Bit Operations/Bitwise Operator  logicop=AND  UseBitMask=off  NumInputPorts=2  BitMask=bin2dec('11011001')  BitMaskRealWorld=Stored Integer
  M1TorqueSet_And1 : simulink/Logic and Bit Operations/Bitwise Operator  logicop=AND  UseBitMask=off  NumInputPorts=2  BitMask=bin2dec('11011001')  BitMaskRealWorld=Stored Integer
  M1TorqueSet_And1_C : Constant  Value=255  OutDataTypeStr=uint32
  M1TorqueSet_And_C : Constant  Value=65535
  M1TorqueSet_Convert : DataTypeConversion  OutDataTypeStr=uint32
  M1TorqueSet_D : Product  Inputs=*/
  M1TorqueSet_D1 : Product  Inputs=*/
  M1TorqueSet_D2 : Product  Inputs=*/
  M1TorqueSet_F : Constant  Value=0.25  OutDataTypeStr=single
  M1TorqueSet_L : simulink/Logic and Bit Operations/Bitwise Operator  logicop=AND  UseBitMask=on  BitMask=262080  BitMaskRealWorld=Stored Integer
  M1TorqueSet_O : Constant  Value=-300  OutDataTypeStr=single
  M1TorqueSet_S : ArithShift  BitShiftNumber=-6
  M1TorqueSet_sat : Saturate  UpperLimit=723.75  LowerLimit=-300
  M1TorqueSet_st : Sum  Inputs=+-
  M1TorqueSetoutput2_C : Constant  Value=256
  M1TorqueSetoutput3_C : Constant  Value=65536
  output1 : Outport
  output2 : Outport  Port=2
  output3 : Outport  Port=3
  output4 : Outport  Port=4
  output5 : Outport  Port=5
  output6 : Outport  Port=6
  output7 : Outport  Port=7
  output8 : Outport  Port=8
  wires:
  M1TorqueSet/1 -> M1TorqueSet_sat/1
  M1TorqueSet_sat/1 -> M1TorqueSet_st/1
  M1TorqueSet_O/1 -> M1TorqueSet_st/2
  M1TorqueSet_st/1 -> M1TorqueSet_D/1
  M1TorqueSet_F/1 -> M1TorqueSet_D/2
  M1TorqueSet_D/1 -> M1TorqueSetRon/1
  M1TorqueSetRon/1 -> M1TorqueSet_S/1
  M1TorqueSet_S/1 -> M1TorqueSet_1sat/1
  M1TorqueSet_1sat/1 -> M1TorqueSet_Convert/1
  M1TorqueSet_Convert/1 -> M1TorqueSet_L/1
  M1TorqueSet_L/1 -> M1TorqueSet_D1/1, M1TorqueSet_And/1, M1TorqueSet_And1/1
  M1TorqueSetoutput3_C/1 -> M1TorqueSet_D1/2
  M1TorqueSet_D1/1 -> M1TorqueSetCOV/1
  M1TorqueSetCOV/1 -> output3/1
  M1TorqueSet_And_C/1 -> M1TorqueSetBitCov/1
  M1TorqueSetBitCov/1 -> M1TorqueSet_And/2
  M1TorqueSet_And/1 -> M1TorqueSet_D2/1
  M1TorqueSetoutput2_C/1 -> M1TorqueSet_D2/2
  M1TorqueSet_D2/1 -> M1TorqueSetCOV1/1
  M1TorqueSetCOV1/1 -> output2/1
  M1TorqueSet_And1_C/1 -> M1TorqueSet_And1/2
  M1TorqueSet_And1/1 -> M1TorqueSetBitCov1/1
  M1TorqueSetBitCov1/1 -> output1/1
  Constant4/1 -> output4/1
  Constant5/1 -> output5/1
  Constant6/1 -> output6/1
  Constant7/1 -> output7/1
  Constant8/1 -> output8/1

== system DDCU_wxt_v02_forA_LabviewV02/OutputSignalProcess/VCU_MCU1/M2Drive ==
  M2Drive : Inport
  Constant{1..4,6..8} (7 alike) : Constant  Value=0  OutDataTypeStr=uint8
  M2DriveRon : Rounding  Operator=round
  M2Drive_1sat : Saturate  UpperLimit=12  LowerLimit=0
  M2Drive_Convert : DataTypeConversion  OutDataTypeStr=uint8
  M2Drive_Convert1 : DataTypeConversion  OutDataTypeStr=uint32
  M2Drive_D : Product  Inputs=*/
  M2Drive_F : Constant  OutDataTypeStr=single
  M2Drive_L : simulink/Logic and Bit Operations/Bitwise Operator  logicop=AND  UseBitMask=on  BitMask=12  BitMaskRealWorld=Stored Integer
  M2Drive_O : Constant  Value=0  OutDataTypeStr=single
  M2Drive_S : ArithShift  BitShiftNumber=-2
  M2Drive_sat : Saturate  UpperLimit=3  LowerLimit=0
  M2Drive_st : Sum  Inputs=+-
  output1 : Outport
  output2 : Outport  Port=2
  output3 : Outport  Port=3
  output4 : Outport  Port=4
  output5 : Outport  Port=5
  output6 : Outport  Port=6
  output7 : Outport  Port=7
  output8 : Outport  Port=8
  wires:
  M2Drive/1 -> M2Drive_sat/1
  M2Drive_sat/1 -> M2Drive_st/1
  M2Drive_O/1 -> M2Drive_st/2
  M2Drive_st/1 -> M2Drive_D/1
  M2Drive_F/1 -> M2Drive_D/2
  M2Drive_D/1 -> M2DriveRon/1
  M2DriveRon/1 -> M2Drive_S/1
  M2Drive_S/1 -> M2Drive_1sat/1
  M2Drive_1sat/1 -> M2Drive_Convert1/1
  M2Drive_Convert1/1 -> M2Drive_L/1
  M2Drive_L/1 -> M2Drive_Convert/1
  M2Drive_Convert/1 -> output5/1
  Constant1/1 -> output1/1
  Constant2/1 -> output2/1
  Constant3/1 -> output3/1
  Constant4/1 -> output4/1
  Constant6/1 -> output6/1
  Constant7/1 -> output7/1
  Constant8/1 -> output8/1

== system DDCU_wxt_v02_forA_LabviewV02/OutputSignalProcess/VCU_MCU1/M2Enable ==
  M2Enable : Inport
  Constant{1..3,5..8} (7 alike) : Constant  Value=0  OutDataTypeStr=uint8
  M2EnableRon : Rounding  Operator=round
  M2Enable_1sat : Saturate  UpperLimit=192  LowerLimit=0
  M2Enable_Convert : DataTypeConversion  OutDataTypeStr=uint8
  M2Enable_Convert1 : DataTypeConversion  OutDataTypeStr=uint32
  M2Enable_D : Product  Inputs=*/
  M2Enable_F : Constant  OutDataTypeStr=single
  M2Enable_L : simulink/Logic and Bit Operations/Bitwise Operator  logicop=AND  UseBitMask=on  BitMask=192  BitMaskRealWorld=Stored Integer
  M2Enable_O : Constant  Value=0  OutDataTypeStr=single
  M2Enable_S : ArithShift  BitShiftNumber=-6
  M2Enable_sat : Saturate  UpperLimit=3  LowerLimit=0
  M2Enable_st : Sum  Inputs=+-
  output1 : Outport
  output2 : Outport  Port=2
  output3 : Outport  Port=3
  output4 : Outport  Port=4
  output5 : Outport  Port=5
  output6 : Outport  Port=6
  output7 : Outport  Port=7
  output8 : Outport  Port=8
  wires:
  M2Enable/1 -> M2Enable_sat/1
  M2Enable_sat/1 -> M2Enable_st/1
  M2Enable_O/1 -> M2Enable_st/2
  M2Enable_st/1 -> M2Enable_D/1
  M2Enable_F/1 -> M2Enable_D/2
  M2Enable_D/1 -> M2EnableRon/1
  M2EnableRon/1 -> M2Enable_S/1
  M2Enable_S/1 -> M2Enable_1sat/1
  M2Enable_1sat/1 -> M2Enable_Convert1/1
  M2Enable_Convert1/1 -> M2Enable_L/1
  M2Enable_L/1 -> M2Enable_Convert/1
  M2Enable_Convert/1 -> output4/1
  Constant1/1 -> output1/1
  Constant2/1 -> output2/1
  Constant3/1 -> output3/1
  Constant5/1 -> output5/1
  Constant6/1 -> output6/1
  Constant7/1 -> output7/1
  Constant8/1 -> output8/1

== system DDCU_wxt_v02_forA_LabviewV02/OutputSignalProcess/VCU_MCU1/M2Mode ==
  M2Mode : Inport
  Constant{1..4,6..8} (7 alike) : Constant  Value=0  OutDataTypeStr=uint8
  M2ModeRon : Rounding  Operator=round
  M2Mode_1sat : Saturate  UpperLimit=3  LowerLimit=0
  M2Mode_Convert : DataTypeConversion  OutDataTypeStr=uint8
  M2Mode_Convert1 : DataTypeConversion  OutDataTypeStr=uint32
  M2Mode_D : Product  Inputs=*/
  M2Mode_F : Constant  OutDataTypeStr=single
  M2Mode_L : simulink/Logic and Bit Operations/Bitwise Operator  logicop=AND  UseBitMask=on  BitMask=3  BitMaskRealWorld=Stored Integer
  M2Mode_O : Constant  Value=0  OutDataTypeStr=single
  M2Mode_S : ArithShift
  M2Mode_sat : Saturate  UpperLimit=3  LowerLimit=0
  M2Mode_st : Sum  Inputs=+-
  output1 : Outport
  output2 : Outport  Port=2
  output3 : Outport  Port=3
  output4 : Outport  Port=4
  output5 : Outport  Port=5
  output6 : Outport  Port=6
  output7 : Outport  Port=7
  output8 : Outport  Port=8
  wires:
  M2Mode/1 -> M2Mode_sat/1
  M2Mode_sat/1 -> M2Mode_st/1
  M2Mode_O/1 -> M2Mode_st/2
  M2Mode_st/1 -> M2Mode_D/1
  M2Mode_F/1 -> M2Mode_D/2
  M2Mode_D/1 -> M2ModeRon/1
  M2ModeRon/1 -> M2Mode_S/1
  M2Mode_S/1 -> M2Mode_1sat/1
  M2Mode_1sat/1 -> M2Mode_Convert1/1
  M2Mode_Convert1/1 -> M2Mode_L/1
  M2Mode_L/1 -> M2Mode_Convert/1
  M2Mode_Convert/1 -> output5/1
  Constant1/1 -> output1/1
  Constant2/1 -> output2/1
  Constant3/1 -> output3/1
  Constant4/1 -> output4/1
  Constant6/1 -> output6/1
  Constant7/1 -> output7/1
  Constant8/1 -> output8/1

== system DDCU_wxt_v02_forA_LabviewV02/OutputSignalProcess/VCU_MCU1/M2SpeedLimit ==
  M2SpeedLimit : Inport
  Constant{1..6} (6 alike) : Constant  Value=0  OutDataTypeStr=uint8
  M2SpeedLimitBitCov : DataTypeConversion  OutDataTypeStr=uint8
  M2SpeedLimitCOV : DataTypeConversion  OutDataTypeStr=uint8
  M2SpeedLimitRon : Rounding  Operator=round
  M2SpeedLimit_1sat : Saturate  UpperLimit=4095  LowerLimit=0
  M2SpeedLimit_And : simulink/Logic and Bit Operations/Bitwise Operator  logicop=AND  UseBitMask=off  NumInputPorts=2  BitMask=bin2dec('11011001')  BitMaskRealWorld=Stored Integer
  M2SpeedLimit_And_C : Constant  Value=255  OutDataTypeStr=uint32
  M2SpeedLimit_Convert : DataTypeConversion  OutDataTypeStr=uint32
  M2SpeedLimit_D : Product  Inputs=*/
  M2SpeedLimit_D1 : Product  Inputs=*/
  M2SpeedLimit_F : Constant  Value=5  OutDataTypeStr=single
  M2SpeedLimit_L : simulink/Logic and Bit Operations/Bitwise Operator  logicop=AND  UseBitMask=on  BitMask=4095  BitMaskRealWorld=Stored Integer
  M2SpeedLimit_O : Constant  Value=0  OutDataTypeStr=single
  M2SpeedLimit_S : ArithShift
  M2SpeedLimit_sat : Saturate  UpperLimit=20475  LowerLimit=0
  M2SpeedLimit_st : Sum  Inputs=+-
  M2SpeedLimitoutput8_C : Constant  Value=256
  output1 : Outport
  output2 : Outport  Port=2
  output3 : Outport  Port=3
  output4 : Outport  Port=4
  output5 : Outport  Port=5
  output6 : Outport  Port=6
  output7 : Outport  Port=7
  output8 : Outport  Port=8
  wires:
  M2SpeedLimit/1 -> M2SpeedLimit_sat/1
  M2SpeedLimit_sat/1 -> M2SpeedLimit_st/1
  M2SpeedLimit_O/1 -> M2SpeedLimit_st/2
  M2SpeedLimit_st/1 -> M2SpeedLimit_D/1
  M2SpeedLimit_F/1 -> M2SpeedLimit_D/2
  M2SpeedLimit_D/1 -> M2SpeedLimitRon/1
  M2SpeedLimitRon/1 -> M2SpeedLimit_S/1
  M2SpeedLimit_S/1 -> M2SpeedLimit_1sat/1
  M2SpeedLimit_1sat/1 -> M2SpeedLimit_Convert/1
  M2SpeedLimit_Convert/1 -> M2SpeedLimit_L/1
  M2SpeedLimit_L/1 -> M2SpeedLimit_D1/1, M2SpeedLimit_And/1
  M2SpeedLimitoutput8_C/1 -> M2SpeedLimit_D1/2
  M2SpeedLimit_D1/1 -> M2SpeedLimitCOV/1
  M2SpeedLimitCOV/1 -> output8/1
  M2SpeedLimit_And_C/1 -> M2SpeedLimit_And/2
  M2SpeedLimit_And/1 -> M2SpeedLimitBitCov/1
  M2SpeedLimitBitCov/1 -> output7/1
  Constant1/1 -> output1/1
  Constant2/1 -> output2/1
  Constant3/1 -> output3/1
  Constant4/1 -> output4/1
  Constant5/1 -> output5/1
  Constant6/1 -> output6/1

== system DDCU_wxt_v02_forA_LabviewV02/OutputSignalProcess/VCU_MCU1/M2TorqueSet ==
  M2TorqueSet : Inport
  Constant{1..4,7..8} (6 alike) : Constant  Value=0  OutDataTypeStr=uint8
  M2TorqueSetBitCov : DataTypeConversion  OutDataTypeStr=uint8
  M2TorqueSetCOV : DataTypeConversion  OutDataTypeStr=uint8
  M2TorqueSetRon : Rounding  Operator=round
  M2TorqueSet_1sat : Saturate  UpperLimit=65520  LowerLimit=0
  M2TorqueSet_And : simulink/Logic and Bit Operations/Bitwise Operator  logicop=AND  UseBitMask=off  NumInputPorts=2  BitMask=bin2dec('11011001')  BitMaskRealWorld=Stored Integer
  M2TorqueSet_And_C : Constant  Value=255  OutDataTypeStr=uint32
  M2TorqueSet_Convert : DataTypeConversion  OutDataTypeStr=uint32
  M2TorqueSet_D : Product  Inputs=*/
  M2TorqueSet_D1 : Product  Inputs=*/
  M2TorqueSet_F : Constant  Value=0.25  OutDataTypeStr=single
  M2TorqueSet_L : simulink/Logic and Bit Operations/Bitwise Operator  logicop=AND  UseBitMask=on  BitMask=65520  BitMaskRealWorld=Stored Integer
  M2TorqueSet_O : Constant  Value=-300  OutDataTypeStr=single
  M2TorqueSet_S : ArithShift  BitShiftNumber=-4
  M2TorqueSet_sat : Saturate  UpperLimit=723.75  LowerLimit=-300
  M2TorqueSet_st : Sum  Inputs=+-
  M2TorqueSetoutput6_C : Constant  Value=256
  output1 : Outport
  output2 : Outport  Port=2
  output3 : Outport  Port=3
  output4 : Outport  Port=4
  output5 : Outport  Port=5
  output6 : Outport  Port=6
  output7 : Outport  Port=7
  output8 : Outport  Port=8
  wires:
  M2TorqueSet/1 -> M2TorqueSet_sat/1
  M2TorqueSet_sat/1 -> M2TorqueSet_st/1
  M2TorqueSet_O/1 -> M2TorqueSet_st/2
  M2TorqueSet_st/1 -> M2TorqueSet_D/1
  M2TorqueSet_F/1 -> M2TorqueSet_D/2
  M2TorqueSet_D/1 -> M2TorqueSetRon/1
  M2TorqueSetRon/1 -> M2TorqueSet_S/1
  M2TorqueSet_S/1 -> M2TorqueSet_1sat/1
  M2TorqueSet_1sat/1 -> M2TorqueSet_Convert/1
  M2TorqueSet_Convert/1 -> M2TorqueSet_L/1
  M2TorqueSet_L/1 -> M2TorqueSet_D1/1, M2TorqueSet_And/1
  M2TorqueSetoutput6_C/1 -> M2TorqueSet_D1/2
  M2TorqueSet_D1/1 -> M2TorqueSetCOV/1
  M2TorqueSetCOV/1 -> output6/1
  M2TorqueSet_And_C/1 -> M2TorqueSet_And/2
  M2TorqueSet_And/1 -> M2TorqueSetBitCov/1
  M2TorqueSetBitCov/1 -> output5/1
  Constant1/1 -> output1/1
  Constant2/1 -> output2/1
  Constant3/1 -> output3/1
  Constant4/1 -> output4/1
  Constant7/1 -> output7/1
  Constant8/1 -> output8/1

== system DDCU_wxt_v02_forA_LabviewV02/OutputSignalProcess/VCU_MCU1/MCU1HeartBeat ==
  MCU1HeartBeat : Inport
  Constant{1..7} (7 alike) : Constant  Value=0  OutDataTypeStr=uint8
  MCU1HeartBeatRon : Rounding  Operator=round
  MCU1HeartBeat_1sat : Saturate  UpperLimit=240  LowerLimit=0
  MCU1HeartBeat_Convert : DataTypeConversion  OutDataTypeStr=uint8
  MCU1HeartBeat_Convert1 : DataTypeConversion  OutDataTypeStr=uint32
  MCU1HeartBeat_D : Product  Inputs=*/
  MCU1HeartBeat_F : Constant  OutDataTypeStr=single
  MCU1HeartBeat_L : simulink/Logic and Bit Operations/Bitwise Operator  logicop=AND  UseBitMask=on  BitMask=240  BitMaskRealWorld=Stored Integer
  MCU1HeartBeat_O : Constant  Value=0  OutDataTypeStr=single
  MCU1HeartBeat_S : ArithShift  BitShiftNumber=-4
  MCU1HeartBeat_sat : Saturate  UpperLimit=15  LowerLimit=0
  MCU1HeartBeat_st : Sum  Inputs=+-
  output1 : Outport
  output2 : Outport  Port=2
  output3 : Outport  Port=3
  output4 : Outport  Port=4
  output5 : Outport  Port=5
  output6 : Outport  Port=6
  output7 : Outport  Port=7
  output8 : Outport  Port=8
  wires:
  MCU1HeartBeat/1 -> MCU1HeartBeat_sat/1
  MCU1HeartBeat_sat/1 -> MCU1HeartBeat_st/1
  MCU1HeartBeat_O/1 -> MCU1HeartBeat_st/2
  MCU1HeartBeat_st/1 -> MCU1HeartBeat_D/1
  MCU1HeartBeat_F/1 -> MCU1HeartBeat_D/2
  MCU1HeartBeat_D/1 -> MCU1HeartBeatRon/1
  MCU1HeartBeatRon/1 -> MCU1HeartBeat_S/1
  MCU1HeartBeat_S/1 -> MCU1HeartBeat_1sat/1
  MCU1HeartBeat_1sat/1 -> MCU1HeartBeat_Convert1/1
  MCU1HeartBeat_Convert1/1 -> MCU1HeartBeat_L/1
  MCU1HeartBeat_L/1 -> MCU1HeartBeat_Convert/1
  MCU1HeartBeat_Convert/1 -> output8/1
  Constant1/1 -> output1/1
  Constant2/1 -> output2/1
  Constant3/1 -> output3/1
  Constant4/1 -> output4/1
  Constant5/1 -> output5/1
  Constant6/1 -> output6/1
  Constant7/1 -> output7/1
